simulink model "US_Image_Acquire_Trigger_V2"  (R2019a)
settings: Solver=FixedStepAuto  StartTime=0.0  StopTime=inf  FixedStep=Sam_time  RelTol=1e-3
values from neighbouring files (symbols this model uses):
  Epiphan_speed = round(1/Epiphan_speed,3)    [Simulink_Image_Acq_V2.m]    (also in Testing_Script.m)
  Sam_time = 0.034    [Simulink_Image_Acq.m]    (also in Simulink_Image_Acq_V2.m = round(1/Sam_time,3))
  Tot_exp_num = 8    [Simulink_Image_Acq.m]    (also in Simulink_Image_Acq_V2.m = 1)
  UDP_in = 12    [Simulink_Image_Acq.m]    (also in Simulink_Image_Acq_V2.m)
undefined symbols (not defined in the file or in its folder): Cur_exp_num, none, videoinput
libraries: powerlib_meascontrol x3, dspnetwork x2, imaqlib x1, sldrtlib x1
(part 1 of 2)
settings Model: EnablePacing=on  Creator=asgar  LastModifiedBy=David
settings DataIOCC: ReturnWorkspaceOutputs=off
settings DebuggingCC: ArithmeticOperatorsInVariantConditions=warning

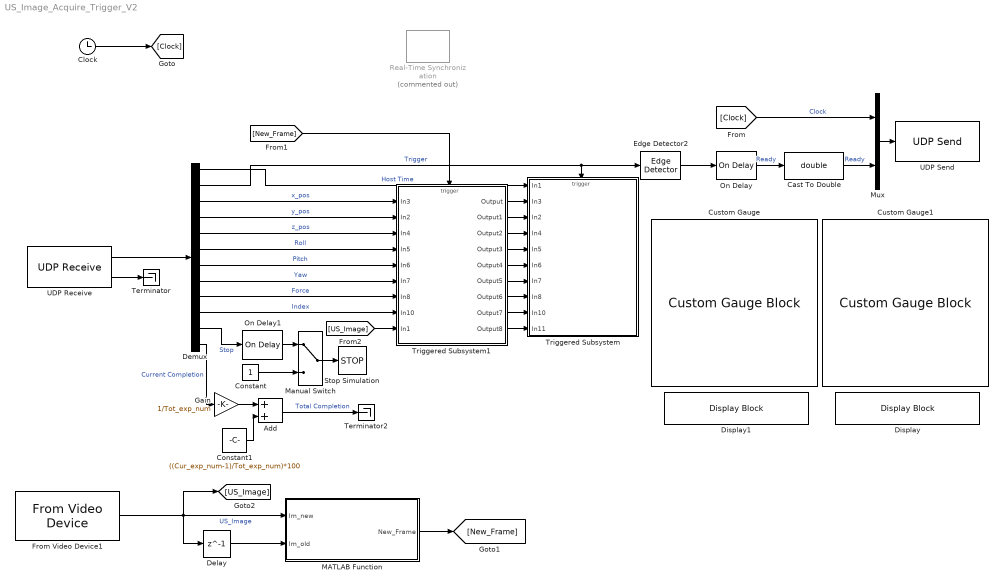
== system US_Image_Acquire_Trigger_V2 ==
  Add : Sum
  Cast To Double : DataTypeConversion  OutDataTypeStr=double
  Clock : Clock
  Constant : Constant
  Constant1 : Constant  Value=((Cur_exp_num-1)/Tot_exp_num)*100  SampleTime=Sam_time
  Custom Gauge : CustomGaugeBlock  NeedleImage=data:image/svg+xml;base64,PD94bWwgdmVyc2lvbj0iMS4wIiBlbmNvZGluZz0idXRmLTgiPz4KPCEtLSBHZW5lcmF0b3I6IEFkb2JlIElsbHVzdHJhdG9yIDE5LjIuMSwgU1ZHIEV4cG9ydCBQbHVnLUluIC4gU1ZHIFZlcnNpb246IDYuMDAgQnVpbGQgMCkgIC0tPgo8c3ZnIHZlcnNpb249IjEuMSIgeG1sbnM9Imh0dHA6Ly93d3cudzMub3JnLzIwMDAvc3ZnIiB4bWxuczp4bGluaz0iaHR0cDovL3d3dy53My5vcmcvMTk5OS94bGluayIgeD0iMHB4IiB5PSIwcHgiCgkgdmlld0JveD0iMCAwIDIwMCA1MCIgc3R5bGU9ImVuYWJsZS1iYWNrZ3JvdW5kOm5ldyAw ...(+9940 chars)  NeedleXPos=0.3802298124325669  NeedleYPos=0.48117305677424654  NeedleHeight=0.11602152693163792  NeedleWidth=0.1911368983686954  NeedleInitialRotation=-59.94322499147643  BackgroundImage=data:image/svg+xml;base64,PD94bWwgdmVyc2lvbj0iMS4wIiBlbmNvZGluZz0iVVRGLTgiIHN0YW5kYWxvbmU9Im5vIj8+CjwhLS0gR2VuZXJhdG9yOiBBZG9iZSBJbGx1c3RyYXRvciAxOS4yLjEsIFNWRyBFeHBvcnQgUGx1Zy1JbiAuIFNWRyBWZXJzaW9uOiA2LjAwIEJ1aWxkIDApICAtLT4KCjxzdmcKICAgeG1sbnM6ZGM9Imh0dHA6Ly9wdXJsLm9yZy9kYy9lbGVtZW50cy8xLjEvIgogICB4bWxuczpjYz0iaHR0cDovL2NyZWF0aXZlY29tbW9ucy5vcmcvbnMjIgogICB4bWxuczpyZGY9Imh0dHA6Ly93d3cudzMub3JnLzE5OTkvMDIvMjItcmRmLXN5bnRh ...(+9660 chars)  GaugeArcDefined=true  GaugeArcRadius=0.1358563990074277  GaugeArcStrokeWidth=0.03972965542329953  GaugeArcRotation=240.5385250290321  GaugeArcRatio=0.8333333333333  GaugeArcTransparency=0  ValueArcColor=#1759b0  GaugeTickColor=#faf5c8  ScaleColorsJSON=[]  fixedAspectRatio=on
  Custom Gauge1 : CustomGaugeBlock  NeedleImage=data:image/svg+xml;base64,PD94bWwgdmVyc2lvbj0iMS4wIiBlbmNvZGluZz0idXRmLTgiPz4KPCEtLSBHZW5lcmF0b3I6IEFkb2JlIElsbHVzdHJhdG9yIDE5LjIuMSwgU1ZHIEV4cG9ydCBQbHVnLUluIC4gU1ZHIFZlcnNpb246IDYuMDAgQnVpbGQgMCkgIC0tPgo8c3ZnIHZlcnNpb249IjEuMSIgeG1sbnM9Imh0dHA6Ly93d3cudzMub3JnLzIwMDAvc3ZnIiB4bWxuczp4bGluaz0iaHR0cDovL3d3dy53My5vcmcvMTk5OS94bGluayIgeD0iMHB4IiB5PSIwcHgiCgkgdmlld0JveD0iMCAwIDIwMCA1MCIgc3R5bGU9ImVuYWJsZS1iYWNrZ3JvdW5kOm5ldyAw ...(+9940 chars)  NeedleXPos=0.3802298124325669  NeedleYPos=0.48117305677424654  NeedleHeight=0.11602152693163792  NeedleWidth=0.1911368983686954  NeedleInitialRotation=-59.94322499147643  BackgroundImage=data:image/svg+xml;base64,PD94bWwgdmVyc2lvbj0iMS4wIiBlbmNvZGluZz0iVVRGLTgiIHN0YW5kYWxvbmU9Im5vIj8+CjwhLS0gR2VuZXJhdG9yOiBBZG9iZSBJbGx1c3RyYXRvciAxOS4yLjEsIFNWRyBFeHBvcnQgUGx1Zy1JbiAuIFNWRyBWZXJzaW9uOiA2LjAwIEJ1aWxkIDApICAtLT4KCjxzdmcKICAgeG1sbnM6ZGM9Imh0dHA6Ly9wdXJsLm9yZy9kYy9lbGVtZW50cy8xLjEvIgogICB4bWxuczpjYz0iaHR0cDovL2NyZWF0aXZlY29tbW9ucy5vcmcvbnMjIgogICB4bWxuczpyZGY9Imh0dHA6Ly93d3cudzMub3JnLzE5OTkvMDIvMjItcmRmLXN5bnRh ...(+9660 chars)  GaugeArcDefined=true  GaugeArcRadius=0.1358563990074277  GaugeArcStrokeWidth=0.03972965542329953  GaugeArcRotation=240.5385250290321  GaugeArcRatio=0.8333333333333  GaugeArcTransparency=0  ValueArcColor=#1759b0  GaugeTickColor=#faf5c8  ScaleColorsJSON=[]  fixedAspectRatio=on
  Delay : Delay  DelayLength=1  InputProcessing=Columns as channels (frame based)  SampleTime=Epiphan_speed
  Demux : Demux  Outputs=UDP_in
  Display : DisplayBlock  LabelPosition=Hide  Format=short
  Display1 : DisplayBlock  LabelPosition=Hide  Format=short
  Edge Detector2 : powerlib_meascontrol/Logic/Edge Detector  model=Rising  ic=0  Ts=Sam_time
      settings: SourceProductName=Simscape Electrical  SourceProductBaseCode=PS
  From Video Device1 : imaqlib/From Video Device  DeviceMenu=winvideo 1 (DVI2USB 3.0 D2S300156)  Device=winvideo 1 (DVI2USB 3.0 D2S300156)  ObjConstructor=videoinput('winvideo', 1)  VideoFormatMenu=RGB565_1280x1024  VideoFormat=RGB565_1280x1024  VideoSource=input1  ROIPosition=[107 366 783 395]  EnableHWTrigger=off  TriggerConfiguration=none/none  SampleTime=0.017  OutputPortsMode=One multidimensional signal  DataType=single  CanDoHWTrigger=no  ReturnedColorSpace=grayscale  BlockHandle=4090.0001  ROIWidth=395  ROIHeight=783  ROIColumn=366  ROIRow=107  EngXMLPath=C:\Program Files\MATLAB\R2019a\toolbox\imaq\imaq\private  DevXMLPath=C:\ProgramData\MATLAB\SupportPackages\R2019a\toolbox\imaq\supportpackages\genericvideo\adaptor\win64  EngLibPath=C:\Program Files\MATLAB\R2019a\toolbox\imaq\imaqblks\imaqmex\win64  ColorSpace=grayscale  BayerSensorAlignment=grbg  ImaqMode=off
      settings: SourceProductName=Image Acquisition Toolbox
  Gain : Gain  Gain=1/Tot_exp_num
  MATLAB Function : MATLAB Function  TreatAsAtomicUnit=on
  Manual Switch : ManualSwitch
  Mux : Mux  Inputs=2
  On Delay : powerlib_meascontrol/Logic/On Delay  DelayType=Off delay  delay=Sam_time*4  ic=0  Ts=Sam_time
      settings: SourceProductName=Simscape Electrical
  On Delay1 : powerlib_meascontrol/Logic/On Delay  DelayType=On delay  delay=5/30  ic=0  Ts=Sam_time
      settings: SourceProductName=Simscape Electrical
  Real-Time Synchronization : sldrtlib/Real-Time Synchronization  Commented=on  SampleTime=Sam_time  MaxMissedTicks=10  ShowMissedTicks=off  YieldWhenWaiting=off
  Stop Simulation : Stop
  Terminator : Terminator
  Terminator2 : Terminator
  Triggered Subsystem : Subsystem  TreatAsAtomicUnit=on
  Triggered Subsystem1 : Subsystem  TreatAsAtomicUnit=on
  UDP Receive : dspnetwork/UDP Receive  localURL='0.0.0.0'  localPort=52050  remoteURL='192.168.0.3'  remotePort=-1  recvBufferSize=UDP_in*8  dims=UDP_in  signalDatatype=double  isComplex=off  isVarSize=off  showBlockingTime=off  blockingTime=0  sampletime=Sam_time  blockPlatform=[]
      settings: SourceProductName=DSP System Toolbox  SourceProductBaseCode=DS
  UDP Send : dspnetwork/UDP Send  remoteURL='192.168.0.3'  remotePort=52051  localURL='0.0.0.0'  localPortSource=Automatically determine  localPort=-1  sampletime=-1  blockPlatform=[]  separateLengthPort=0
      settings: SourceProductName=Simulink
  wires:
  UDP Receive/1 -> Demux/1
  Demux/2 -> Triggered Subsystem/Trigger, Edge Detector2/1  "Trigger"
  Demux/1 -> Triggered Subsystem/1(In1)  "Host Time"
  Demux/11 -> On Delay1/1  "Stop"
  Mux/1 -> UDP Send/1
  Clock/1 -> [Clock]
  [Clock] -> Mux/1  "Clock"
  On Delay/1 -> Cast To Double/1  "Ready"
  Cast To Double/1 -> Mux/2  "Ready"
  UDP Receive/2 -> Terminator/1
  Edge Detector2/1 -> On Delay/1
  On Delay1/1 -> Manual Switch/1
  Manual Switch/1 -> Stop Simulation/1
  Constant/1 -> Manual Switch/2
  Demux/12 -> Gain/1  "Current Completion"
  Gain/1 -> Add/1
  Constant1/1 -> Add/2
  Add/1 -> Terminator2/1  "Total Completion"
  Delay/1 -> MATLAB Function/2(Im_old)
  From Video Device1/1 -> [US_Image], MATLAB Function/1(Im_new), Delay/1  "US_Image"
  MATLAB Function/1(New_Frame) -> [New_Frame]
  [New_Frame] -> Triggered Subsystem1/Trigger
  Triggered Subsystem1/1(Output) -> Triggered Subsystem/2(In3)
  Triggered Subsystem1/2(Output1) -> Triggered Subsystem/3(In2)
  Triggered Subsystem1/3(Output2) -> Triggered Subsystem/4(In4)
  Triggered Subsystem1/4(Output3) -> Triggered Subsystem/5(In5)
  Triggered Subsystem1/5(Output4) -> Triggered Subsystem/6(In6)
  Triggered Subsystem1/6(Output5) -> Triggered Subsystem/7(In7)
  Triggered Subsystem1/7(Output6) -> Triggered Subsystem/8(In8)
  Triggered Subsystem1/8(Output7) -> Triggered Subsystem/9(In10)
  Triggered Subsystem1/9(Output8) -> Triggered Subsystem/10(In11)
  Demux/3 -> Triggered Subsystem1/1(In3)  "x_pos"
  Demux/4 -> Triggered Subsystem1/2(In2)  "y_pos"
  Demux/5 -> Triggered Subsystem1/3(In4)  "z_pos"
  Demux/6 -> Triggered Subsystem1/4(In5)  "Roll"
  Demux/7 -> Triggered Subsystem1/5(In6)  "Pitch"
  Demux/8 -> Triggered Subsystem1/6(In7)  "Yaw"
  Demux/9 -> Triggered Subsystem1/7(In8)  "Force"
  Demux/10 -> Triggered Subsystem1/8(In10)  "Index"
  [US_Image] -> Triggered Subsystem1/9(In1)

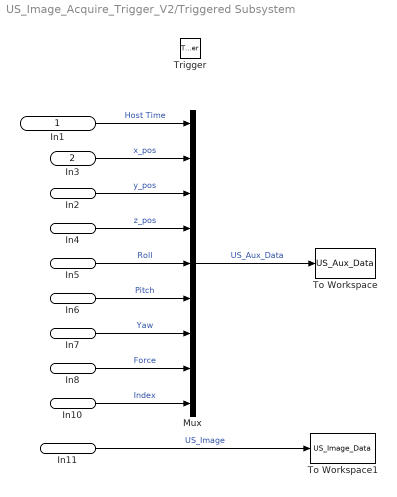
== system US_Image_Acquire_Trigger_V2/Triggered Subsystem ==
  In1 : Inport
  In3 : Inport  Port=2
  In2 : Inport  Port=3
  In4 : Inport  Port=4
  In5 : Inport  Port=5
  In6 : Inport  Port=6
  In7 : Inport  Port=7
  In8 : Inport  Port=8
  In10 : Inport  Port=9
  In11 : Inport  Port=10
  Trigger : TriggerPort  VariantControl=Variant
  Mux : Mux  Inputs=9
  To Workspace : ToWorkspace  VariableName=US_Aux_Data  SampleTime=-1
      settings: Save2DSignal=2-D array (concatenate along first dimension)
  To Workspace1 : ToWorkspace  VariableName=US_Image_Data  SaveFormat=Structure With Time  SampleTime=-1
      settings: Save2DSignal=2-D array (concatenate along first dimension)
  wires:
  In1/1 -> Mux/1  "Host Time"
  In3/1 -> Mux/2  "x_pos"
  In2/1 -> Mux/3  "y_pos"
  In4/1 -> Mux/4  "z_pos"
  In5/1 -> Mux/5  "Roll"
  In6/1 -> Mux/6  "Pitch"
  In7/1 -> Mux/7  "Yaw"
  In8/1 -> Mux/8  "Force"
  Mux/1 -> To Workspace/1  "US_Aux_Data"
  In10/1 -> Mux/9  "Index"
  In11/1 -> To Workspace1/1  "US_Image"

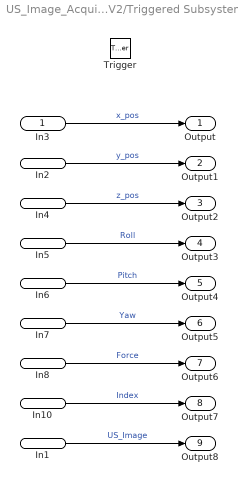
== system US_Image_Acquire_Trigger_V2/Triggered Subsystem1 ==
  In3 : Inport
  In2 : Inport  Port=2
  In4 : Inport  Port=3
  In5 : Inport  Port=4
  In6 : Inport  Port=5
  In7 : Inport  Port=6
  In8 : Inport  Port=7
  In10 : Inport  Port=8
  In1 : Inport  Port=9
  Trigger : TriggerPort  VariantControl=Variant
  Output : Outport
  Output1 : Outport  Port=2
  Output2 : Outport  Port=3
  Output3 : Outport  Port=4
  Output4 : Outport  Port=5
  Output5 : Outport  Port=6
  Output6 : Outport  Port=7
  Output7 : Outport  Port=8
  Output8 : Outport  Port=9
  wires:
  In3/1 -> Output/1  "x_pos"
  In2/1 -> Output1/1  "y_pos"
  In4/1 -> Output2/1  "z_pos"
  In5/1 -> Output3/1  "Roll"
  In6/1 -> Output4/1  "Pitch"
  In7/1 -> Output5/1  "Yaw"
  In8/1 -> Output6/1  "Force"
  In10/1 -> Output7/1  "Index"
  In1/1 -> Output8/1  "US_Image"
